simulink model "sldemo_radar_eml"  (Simulink 7.6)
settings: Solver=ode5  SolverMode=SingleTasking  StartTime=0.0  StopTime=100  FixedStep=0.1  MaxStep=0.1  RelTol=1e-3  AbsTol=1e-6
StartFcn:
  | clear radarLogsOut
StopFcn:
  | aero_radplot;
model workspace (MATLAB code in the model file):
  | g = 32.2;    % Acceleration due to gravity (ft/sec^2)
  | tauc = 5;    % Correlation time of aircraft cross axis acceleration
  | tauT = 4;    % Correlation time of aircraft thrust axis acceleration
  | Speed = 400; % Initial speed of aircraft in y direction feet/sec
  | deltat = 1;  % Radar update rate (also hard-coded in extkalman.m)
libraries: simulink x2
Description:
  | Radar Tracking Using Embedded MATLAB(R)
  | 
  | This demonstration shows how to use an extended Kalman filter with the
  | Embedded MATLAB(R) Function block in Simulink(R) to estimate an aircraft's
  | position from radar measurements. The filter implementation is found in the
  | Embedded MATLAB Function block, the contents of which are stored in the
  | Simulink model itself.
  | 
  | At the end of the simulation, three figures display the following information: the
  | actual trajectory compared to the estimated trajectory; the estimation residual
  | for range; and the actual, measured, and estimated positions.
CloseFcn:
  | h=findobj('type','figure');if ~isempty(h);close(h);end
  | clear radarLogsOut
settings Model: Creator=The MathWorks Inc.  CovMetricSettings=d  ExtModeTrigMode=oneshot  ExtModeArmWhenConnect=off  ExtModeAutoUpdateStatusClock=off
settings DataIOCC: LimitDataPoints=off  SaveOutput=off  SaveTime=off  TimeSaveName=t_sim  SignalLoggingName=radarLogsOut
settings OptimizationCC: InlineParams=on  InlineInvariantSignals=on  StateBitsets=on  DataBitsets=on  UseTempVars=on  ZeroExternalMemoryAtStartup=off  ZeroInternalMemoryAtStartup=off  NoFixptDivByZeroProtection=on  OptimizeModelRefInitCode=on  LifeSpan=1  BufferReusableBoundary=off
settings DebuggingCC: SaveWithParameterizedLinksMsg=none  CheckExecutionContextPreStartOutputMsg=on  CheckExecutionContextRuntimeOutputMsg=on  SignalResolutionControl=TryResolveAllWithWarning  SolverPrmCheckMsg=none  MultiTaskDSMMsg=warning  MultiTaskCondExecSysMsg=none
settings SFSimCC: SimParseCustomCode=off
settings RTWCC: SystemTargetFile=ert.tlc  TLCOptions=-p0 -aWarnNonSaturatedBlocks=0  TemplateMakefile=ert_default_tmf  Description=RTW Embedded Coder (no auto configuration)  GenerateReport=on  RTWVerbose=off  ProcessScript=ert_make_rtw_hook  IncludeHyperlinkInReport=on  LaunchReport=on  IncludeERTFirstTime=on
settings CodeAppCC: ForceParamTrailComments=on  IgnoreCustomStorageClasses=off  SimulinkDataObjDesc=on  CustomSymbolStrFcn=$F$N$M  CustomSymbolStrMacro=$N$M  InsertBlockDesc=on
settings ERTTargetCC: TargetFcnLib=ansi_tfl_tmw.mat  MultiwordLength=2048  GenerateSampleERTMain=on  IncludeMdlTerminateFcn=off  SupportComplex=off  SupportContinuousTime=on  SupportNonInlinedSFcns=on  InlinedParameterPlacement=NonHierarchical  ERTCustomFileTemplate=example_file_process.tlc  ConvertIfToSwitch=off

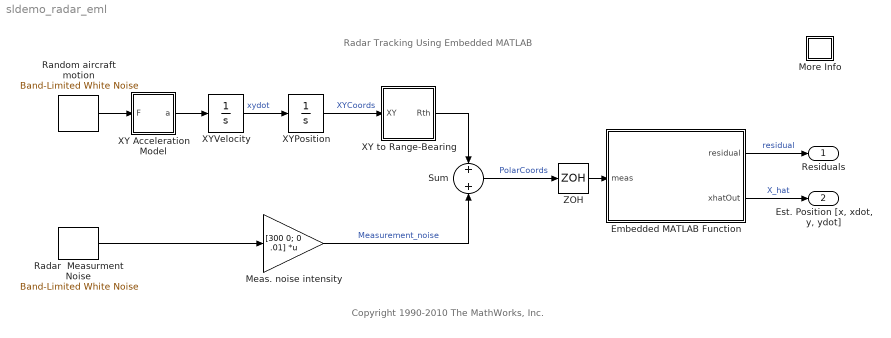
== system sldemo_radar_eml ==
  note: Radar Tracking Using Embedded MATLAB
  note: Copyright 1990-2010 The MathWorks, Inc.
  Embedded MATLAB Function : Stateflow chart  TreatAsAtomicUnit=on
  Meas. noise intensity : Gain  Gain=[300 0; 0 .01]  Multiplication=Matrix(K*u) (u vector)
  More Info : Subsystem
      settings: OpenFcn=showdemo(bdroot(gcs))
      mask Display: disp('?')
  Radar  Measurment Noise : simulink/Sources/Band-Limited White Noise  SystemSampleTime=-1  Cov=[1 1]  Ts=0.1  seed=[52341 62341]
  Random aircraft motion : simulink/Sources/Band-Limited White Noise  SystemSampleTime=-1  Cov=[0.001 .001]  Ts=0.1  seed=[58413 74925]
  Sum : Sum  Inputs=2  SaturateOnIntegerOverflow=on  InputSameDT=on  OutDataTypeStr=Inherit: Same as first input
  XY Acceleration Model : Subsystem
  XY to Range-Bearing : Subsystem
      mask Type: xy2rtheta
      mask Description:
      | Vector transformation from cartesian to polar coordinates.
      | input:   [x, y]
      | output: [r, theta]
      | 
      | r = hypot(x,y));
      | theta = atan2(y,x);
      mask Help: Use "Look under mask" to see the implementation, done in Simulink blocks.
      mask Display: plot(0,0,100,100,[24,20,15,20,20],[85,95,85,95,20],[80,20,95,85,95,85],[70,20,20,15,20,24],[56,56,55,52,50,46],[20,26,31,35,38,42])
  XYPosition : Integrator
  XYVelocity : Integrator  InitialCondition=[0, Speed]
  ZOH : ZeroOrderHold  SampleTime=deltat
  Residuals : Outport
  "Est. Position [x, xdot, y, ydot]" : Outport  Port=2
  wires:
  XYPosition/1 -> XY to Range-Bearing/1(XY)  "XYCoords"
  XY to Range-Bearing/1(Rth) -> Sum/1
  Sum/1 -> ZOH/1  "PolarCoords"
  XYVelocity/1 -> XYPosition/1  "xydot"
  XY Acceleration Model/1(a) -> XYVelocity/1
  Embedded MATLAB Function/1(residual) -> Residuals/1  "residual"
  Random aircraft motion/1 -> XY Acceleration Model/1(F)
  Embedded MATLAB Function/2(xhatOut) -> "Est. Position [x, xdot, y, ydot]"/1  "X_hat"
  Radar  Measurment Noise/1 -> Meas. noise intensity/1
  Meas. noise intensity/1 -> Sum/2  "Measurement_noise"
  ZOH/1 -> Embedded MATLAB Function/1(meas)

== system sldemo_radar_eml/More Info ==

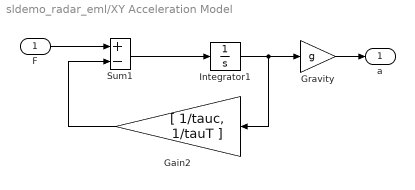
== system sldemo_radar_eml/XY Acceleration Model ==
  F : Inport
  Gain2 : Gain  Gain=[ 1/tauc, 1/tauT ]  SaturateOnIntegerOverflow=on  OutDataTypeStr=Inherit: Same as input  ParamDataTypeStr=Inherit: Same as input
  Gravity : Gain  Gain=g  SaturateOnIntegerOverflow=on  OutDataTypeStr=Inherit: Same as input  ParamDataTypeStr=Inherit: Same as input
  Integrator1 : Integrator
  Sum1 : Sum  Inputs=+-  SaturateOnIntegerOverflow=on  InputSameDT=on  OutDataTypeStr=Inherit: Same as first input
  a : Outport  InitialOutput=0
  wires:
  F/1 -> Sum1/1
  Gain2/1 -> Sum1/2
  Integrator1/1 -> Gravity/1, Gain2/1
  Sum1/1 -> Integrator1/1
  Gravity/1 -> a/1

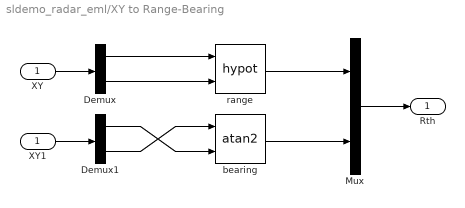
== system sldemo_radar_eml/XY to Range-Bearing ==
  XY : Inport
  Demux : Demux  Outputs=2
  Demux1 : Demux  Outputs=2
  Mux : Mux  Inputs=2
  XY1 : InportShadow  Port=1
  bearing : Trigonometry  Operator=atan2
  range : Math  Operator=hypot  SaturateOnIntegerOverflow=on
  Rth : Outport  InitialOutput=0
  wires:
  Mux/1 -> Rth/1
  range/1 -> Mux/1
  XY/1 -> Demux/1
  Demux/1 -> range/1
  Demux/2 -> range/2
  XY1/1 -> Demux1/1
  bearing/1 -> Mux/2
  Demux1/1 -> bearing/2
  Demux1/2 -> bearing/1

== matlab function Embedded MATLAB Function ==
  data: meas input double; residual output double; deltat parameter double; xhatOut output double
function [residual, xhatOut] = EXTKALMAN(meas, deltat)
%EXTKALMAN Radar Data Processing Tracker Using an Extended Kalman Filter
%
%  This program is executed as a MATLAB function block in the 
%  aero_radmod Simulink model.  There is a file called "aero_raddat.m" that 
%  contains the data needed to run the aero_radmod model.  The estimated 
%  and actual positions are saved to the workspace and are plotted at
%  the end of the simulation by the program aero_radplot (called from the 
%  simulation automatically).
%
%  See the description in the "Extended Kalman Filter" Brochure for 
%  the equations.

%  This program was developed by Dr. Richard Gran, September 1, 1996, 
%  and modified by Paul Barnard, June 1997.
%  Copyright 1990-2009 The MathWorks, Inc.
%  $Revision: 1.1.6.8 $  $Date: 2010/05/20 03:16:17 $


% Initialization
persistent P;
persistent xhat
if isempty(P)
    xhat = [0.001; 0.01; 0.001; 400];
    P = zeros(4);
end
    
%  Radar update time deltat is inherited from model workspace

% 1. Compute Phi, Q, and R 
Phi = [1 deltat 0 0; 0 1 0 0 ; 0 0 1 deltat; 0 0 0 1];
Q =  diag([0 .005 0 .005]);
R =  diag([300^2 0.001^2]);

% 2. Propagate the covariance matrix:
P = Phi*P*Phi' + Q;

% 3. Propagate the track estimate::
xhat = Phi*xhat;

% 4 a). Compute observation estimates:
Rangehat = sqrt(xhat(1)^2+xhat(3)^2);
Bearinghat = atan2(xhat(3),xhat(1));

% 4 b). Compute observation vector y and linearized measurement matrix M 
yhat = 	[Rangehat;
          Bearinghat];
M = [ cos(Bearinghat)          0 sin(Bearinghat)          0
   -sin(Bearinghat)/Rangehat 0 cos(Bearinghat)/Rangehat 0 ];

% 4 c).  Compute residual (Estimation Error)
residual = meas - yhat;

% 5. Compute Kalman Gain:
W = P*M'*inv(M*P*M'+ R);

% 6. Update estimate
xhat = xhat + W*residual;

% 7. Update Covariance Matrix
P = (eye(4)-W*M)*P*(eye(4)-W*M)' + W*R*W';

xhatOut = xhat;
